simulink subsystem "PvtSubSys_VSM_ACC"  (R2020b)
settings: Solver=VariableStepAuto  StartTime=0.0  StopTime=10.0  RelTol=1e-3
values from neighbouring files (symbols this model uses):
  P_VSM_ACC_AutoGoSW = 1.0    [ACC.sldd]
  P_VSM_ACC_BOMEntry_ACCDecReqValue = -0.5    [ACC.sldd]
  P_VSM_ACC_BOMEntry_AxvRefMs2 = -0.5    [ACC.sldd]
  P_VSM_ACC_BOMExit_ACCDecReqValue = -0.3    [ACC.sldd]
  P_VSM_ACC_BrakeOnlyNum = 500.0    [ACC.sldd]
  P_VSM_ACC_RadarOffset = 0.5    [ACC.sldd]
  P_VSM_ACC_StandActiveNumACCMode = 1500.0    [ACC.sldd]
  P_VSM_ACC_StandActiveNumHWAMode = 1500.0    [ACC.sldd]
  P_VSM_ACCExit_AccOverride = 900.0    [ACC.sldd]
  P_VSM_ACCExit_StandWaitTime = 180.0    [ACC.sldd]
  P_VSM_TJA_ActiveWaitNum = 3000.0    [ACC.sldd]
undefined symbols (not defined in the file or in its folder): ACC_STATE, HWAError_Error, HWAError_ErrorBlindness, HWAError_ErrorFast, HWAError_Inhibit, P_Global_VehiclePowerType, P_VSM_PowerTrainConfig, TJA_STATE
libraries: simulink x136, TrueDurationTime x17
(part 1 of 2)
settings Model: Creator=GW00133806  LastModifiedBy=GW00201299

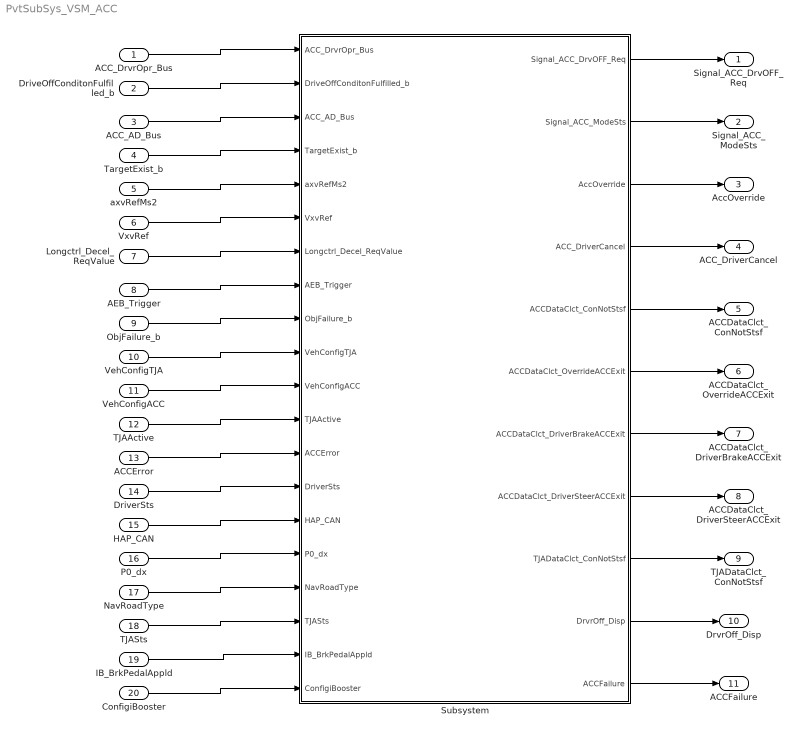
== system PvtSubSys_VSM_ACC ==
  ACC_DrvrOpr_Bus : Inport  OutDataTypeStr=Bus: ACC_DrvrOpr_Bus
  DriveOffConditonFulfilled_b : Inport  Port=2  OutDataTypeStr=boolean
  ACC_AD_Bus : Inport  Port=3
  TargetExist_b : Inport  Port=4  OutDataTypeStr=boolean
  axvRefMs2 : Inport  Port=5  OutDataTypeStr=single
  VxvRef : Inport  Port=6  OutDataTypeStr=single
  Longctrl_Decel_ReqValue : Inport  Port=7  OutDataTypeStr=single
  AEB_Trigger : Inport  Port=8  OutDataTypeStr=boolean
  ObjFailure_b : Inport  Port=9  OutDataTypeStr=boolean
  VehConfigTJA : Inport  Port=10  OutDataTypeStr=boolean
  VehConfigACC : Inport  Port=11  OutDataTypeStr=boolean
  TJAActive : Inport  Port=12  OutDataTypeStr=boolean
  ACCError : Inport  Port=13  OutDataTypeStr=uint8
  DriverSts : Inport  Port=14  OutDataTypeStr=uint8
  HAP_CAN : Inport  Port=15  OutDataTypeStr=Bus: HAP_CAN
  P0_dx : Inport  Port=16  OutDataTypeStr=single
  NavRoadType : Inport  Port=17  OutDataTypeStr=uint8
  TJASts : Inport  Port=18
  IB_BrkPedalAppld : Inport  Port=19
  ConfigiBooster : Inport  Port=20
  Subsystem : Subsystem
  Signal_ACC_DrvOFF_Req : Outport
  Signal_ACC_ModeSts : Outport  Port=2
  AccOverride : Outport  Port=3
  ACC_DriverCancel : Outport  Port=4
  ACCDataClct_ConNotStsf : Outport  Port=5
  ACCDataClct_OverrideACCExit : Outport  Port=6
  ACCDataClct_DriverBrakeACCExit : Outport  Port=7
  ACCDataClct_DriverSteerACCExit : Outport  Port=8
  TJADataClct_ConNotStsf : Outport  Port=9
  DrvrOff_Disp : Outport  Port=10
  ACCFailure : Outport  Port=11
  wires:
  ConfigiBooster/1 -> Subsystem/20(ConfigiBooster)
  IB_BrkPedalAppld/1 -> Subsystem/19(IB_BrkPedalAppld)
  NavRoadType/1 -> Subsystem/17(NavRoadType)
  Subsystem/9(TJADataClct_ConNotStsf) -> TJADataClct_ConNotStsf/1
  Subsystem/4(ACC_DriverCancel) -> ACC_DriverCancel/1
  Subsystem/6(ACCDataClct_OverrideACCExit) -> ACCDataClct_OverrideACCExit/1
  VxvRef/1 -> Subsystem/6(VxvRef)
  Subsystem/7(ACCDataClct_DriverBrakeACCExit) -> ACCDataClct_DriverBrakeACCExit/1
  TargetExist_b/1 -> Subsystem/4(TargetExist_b)
  TJAActive/1 -> Subsystem/12(TJAActive)
  Subsystem/8(ACCDataClct_DriverSteerACCExit) -> ACCDataClct_DriverSteerACCExit/1
  Longctrl_Decel_ReqValue/1 -> Subsystem/7(Longctrl_Decel_ReqValue)
  axvRefMs2/1 -> Subsystem/5(axvRefMs2)
  Subsystem/5(ACCDataClct_ConNotStsf) -> ACCDataClct_ConNotStsf/1
  VehConfigTJA/1 -> Subsystem/10(VehConfigTJA)
  Subsystem/1(Signal_ACC_DrvOFF_Req) -> Signal_ACC_DrvOFF_Req/1
  ACCError/1 -> Subsystem/13(ACCError)
  Subsystem/3(AccOverride) -> AccOverride/1
  VehConfigACC/1 -> Subsystem/11(VehConfigACC)
  Subsystem/2(Signal_ACC_ModeSts) -> Signal_ACC_ModeSts/1
  ObjFailure_b/1 -> Subsystem/9(ObjFailure_b)
  AEB_Trigger/1 -> Subsystem/8(AEB_Trigger)
  ACC_DrvrOpr_Bus/1 -> Subsystem/1(ACC_DrvrOpr_Bus)
  DriveOffConditonFulfilled_b/1 -> Subsystem/2(DriveOffConditonFulfilled_b)
  ACC_AD_Bus/1 -> Subsystem/3(ACC_AD_Bus)
  DriverSts/1 -> Subsystem/14(DriverSts)
  HAP_CAN/1 -> Subsystem/15(HAP_CAN)
  P0_dx/1 -> Subsystem/16(P0_dx)
  Subsystem/10(DrvrOff_Disp) -> DrvrOff_Disp/1
  Subsystem/11(ACCFailure) -> ACCFailure/1
  TJASts/1 -> Subsystem/18(TJASts)

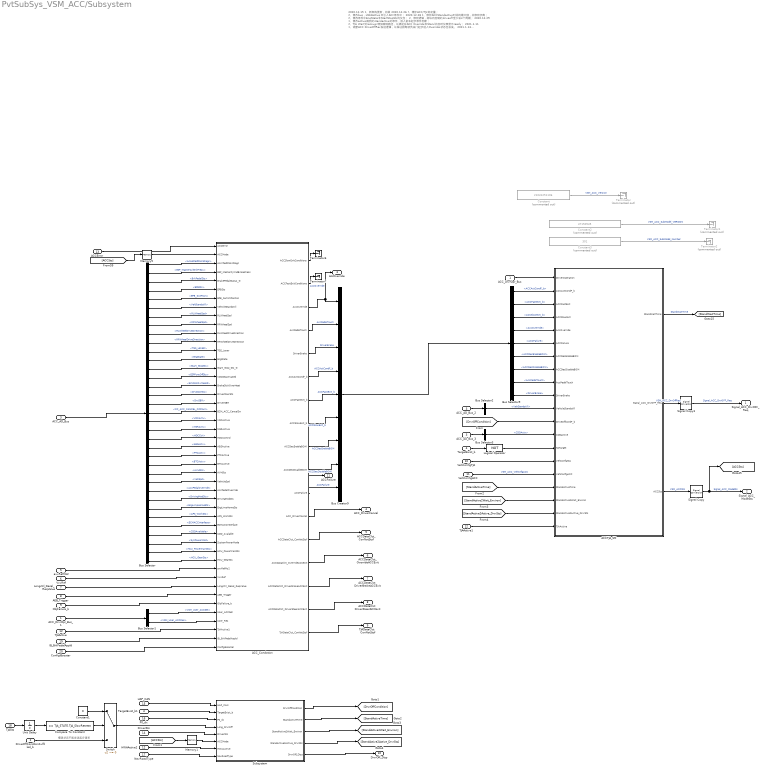
== system PvtSubSys_VSM_ACC/Subsystem ==
  note: 2020.12.15
      | 1、新架构更新，初版
      | 2020.12.26
      | 1、增加ACC/TJA标定量；
      | 2、修改bug，HWAActive未引入ACC条件中；
      | 2020.12.28
      | 1、修改ACCStandactive时间的最大值，并修改字典；
      | 2、修改条件中EngState和StartStopSts的交互；
      | 3、修改逻辑，给纵向控制的driveoff至少发3个周期；
      | 2020.12.29
      | 1、修改active跳到的standactive的条件，加入前车起步条件判断；
      | 2、TJA_Wait到recover增加跳转路径，以满足在ACC Override和Stand状态时仪表显示ready；
      | 2021.1.11
      | 1、调整ACC DriveOffReq发送逻辑，以保证因驾驶员油门起步进入Override状态也会发。
      | 2021.1.13
      | 添加基于驾驶员状态的自动起步逻辑，并用标定量默认关闭；
      | 2021.1.19
      | ACC起步条件增加；
      | 增加观测量；
      | 2021.1.23
      | TJA状态机修改；
      | 2021.1.25
      | ACC状态机中进入standactive的条件删去driveroff；
      | 2021.1.27
      | 1、TJA进入ready修改；
      | 2、ACCdriveroff修改；
      | 2021.1.30
      | TJA逻辑修改
      | 2021.2.1
      | ACC刹车&&standstill激活条件修改；
      | 2021.2.2
      | TJA override逻辑加入HWAActive判断；
      | 2021.2.3
      | TJAWait状态计时bug修改；
      | ACC发DrvrOff逻辑修改；
      | TJAActiveNum阈值修改为4；
      | 2021.2.4
      | DrvrOffReq输出逻辑修改；
      | 2021.2.5
      | ACC Passive状态重写TJAstopexit的值
      | 2021.2.7
      | 增加观测量Override退出条件；
      | 20210217
      | ACCError策略修改；
      | 20210219
      | 删去ACC的CDD和ECM导致的Error，因为在诊断里已经做了，报inhibit
      | 20210224
      | ACC启停条件修改：or2and；
      | 20210308
      | 删去状态机中起步HWA相关条件；
      | 2021.3.12
      | SafeStop置位延迟5s
      | 2021.3.15
      | ACC Override不退出TJA控制；
  note: 慢退状态不能发送起步请求
  ACC_DrvrOpr_Bus : Inport  OutDataTypeStr=Bus: ACC_DrvrOpr_Bus
  DriveOffConditonFulfilled_b : Inport  Port=2  OutDataTypeStr=boolean
  ACC_AD_Bus : Inport  Port=3
  TargetExist_b : Inport  Port=4  OutDataTypeStr=boolean
  axvRefMs2 : Inport  Port=5  OutDataTypeStr=single
  VxvRef : Inport  Port=6  OutDataTypeStr=single
  Longctrl_Decel_ReqValue : Inport  Port=7  OutDataTypeStr=single
  AEB_Trigger : Inport  Port=8  OutDataTypeStr=boolean
  ObjFailure_b : Inport  Port=9  OutDataTypeStr=boolean
  VehConfigTJA : Inport  Port=10  OutDataTypeStr=boolean
  VehConfigACC : Inport  Port=11  OutDataTypeStr=boolean
  TJAActive : Inport  Port=12  OutDataTypeStr=boolean
  ACCError : Inport  Port=13  OutDataTypeStr=uint8
  DriverSts : Inport  Port=14  OutDataTypeStr=uint8
  HAP_CAN : Inport  Port=15  OutDataTypeStr=Bus: HAP_CAN
  P0_dx : Inport  Port=16  OutDataTypeStr=single
  NavRoadType : Inport  Port=17
  TJASts : Inport  Port=18
  IB_BrkPedalAppld : Inport  Port=19
  ConfigiBooster : Inport  Port=20
  ACCTJA_SM : Subsystem
  ACC_AD_Bus_2 : InportShadow  Port=3
  ACC_AD_Bus_3 : InportShadow  Port=3
  ACC_Condotion : Subsystem
  ACC_DrvrOpr_Bus_1 : InportShadow  OutDataTypeStr=Bus: ACC_DrvrOpr_Bus
  Bus Creator9 : BusCreator  Inputs=9
  Bus Selector : BusSelector  OutputSignals=AccelPedlPosnDiagc,ESP_MasterCylBrkPress,BrkPedalSts,EPBSts,EPB_SwtPosn,VehStandstill,RLWheelSpd,RRWheelSpd,RLWheelDriveDirection,RRWheelDriveDirection,TGS_LEVER,EngState,Start_StopSts,ESPFuncOffSts,BrkDskOvrheatd,DrvDoorSts,DrvSBR,CC_ACC_CANCEL_OFFSwt,VDCActv,MSRActv,HDCCtrl,ABSActv,PTCActv,BTCActv,AVHSts,VehSpd,AccPedalOverride,DrivingModDis,EngLimpHomeSts,APS_WorkSts,ECMACCInterface,CDDAvailable,SysPowerMod,HCU_PowertrainSts,HCU_GearSts
  Bus Selector1 : BusSelector  OutputSignals=VSM_User_ACCSet,VSM_User_ACCRes
  Bus Selector2 : BusSelector  OutputSignals=VehStandstill
  Bus Selector3 : BusSelector  OutputSignals=CDDActv
  Bus Selector9 : BusSelector  OutputSignals=ACCActCondF_b,ACCFastExit_b,ACCSlowExit_b,AccOverride,ACCFailure,ACCDecEnableBOM,ACCDecDisableBOM,AccPedalTouch,DriverBrake
  Compare To Constant : simulink/Logic and Bit Operations/Compare To Constant  relop===  const=TJA_STATE.TJA_SlowRetreat  OutDataTypeStr=boolean
  Constant : Constant  Commented=on  Value=21031251106
  Constant1 : Constant  Value=0  OutDataTypeStr=boolean
  Constant2 : Constant  Commented=on  Value=37150535  OutDataTypeStr=uint32
  Constant3 : Constant  Commented=on  Value=301  OutDataTypeStr=uint16
  HWAActive2 : InportShadow  Port=12  OutDataTypeStr=boolean
  Logical Operator : Logic  Operator=NOT  AllPortsSameDT=off  OutDataTypeStr=boolean
  Memory1 : Memory  InitialCondition=ACC_STATE.ACC_Off  InheritSampleTime=on
  Memory5 : Memory  InitialCondition=ACC_STATE.ACC_Off  InheritSampleTime=on
  Signal Copy : SignalConversion  OverrideOpt=off
  Signal Copy3 : SignalConversion  OverrideOpt=off
  Subsystem : Subsystem
  Switch : Switch  Criteria=u2 ~= 0
  TJAActive1 : InportShadow  Port=12  OutDataTypeStr=boolean
  TargetExist_b1 : InportShadow  Port=4  OutDataTypeStr=boolean
  Terminator : Terminator  Commented=on
  Terminator1 : Terminator  Commented=on
  Terminator2 : Terminator  Commented=on
  Terminator6 : Terminator
  Terminator7 : Terminator
  Unit Delay : UnitDelay  InitialCondition=TJA_STATE.TJA_Off  SampleTime=-1  HasFrameUpgradeWarning=on
  Signal_ACC_DrvOFF_Req : Outport
  Signal_ACC_ModeSts : Outport  Port=2
  AccOverride : Outport  Port=3
  ACC_DriverCancel : Outport  Port=4
  ACCDataClct_ConNotStsf : Outport  Port=5
  ACCDataClct_OverrideACCExit : Outport  Port=6
  ACCDataClct_DriverBrakeACCExit : Outport  Port=7
  ACCDataClct_DriverSteerACCExit : Outport  Port=8
  TJADataClct_ConNotStsf : Outport  Port=9
  DrvrOff_Disp : Outport  Port=10
  ACCFailure : Outport  Port=11
  wires:
  Constant2/1 -> Terminator1/1  "VSM_ACC_SubModel_VERSION"
  Constant3/1 -> Terminator2/1  "VSM_ACC_SubModel_Number"
  Switch/1 -> Subsystem/4(Long_DrvrOff)
  Constant1/1 -> Switch/1
  Compare To Constant/1 -> Switch/2
  TJASts/1 -> Unit Delay/1
  TJAActive1/1 -> ACCTJA_SM/20(TJAActive)
  [StandActive2Active_DrvrSts] -> ACCTJA_SM/19(StandActive2Active_DrvrSts)
  [StandActive2Wait_Environ] -> ACCTJA_SM/18(StandActive2Wait_Environ)
  [StandActiveTime] -> ACCTJA_SM/17(StandActiveTime)
  Subsystem/5(DrvrOff_Disp) -> DrvrOff_Disp/1
  Subsystem/4(StandActive2Active_DrvrSts) -> [StandActive2Active_DrvrSts]
  Subsystem/3(StandActive2Wait_Environ) -> [StandActive2Wait_Environ]
  Subsystem/2(StandActiveTime) -> [StandActiveTime]
  NavRoadType/1 -> Subsystem/8(NavRoadType)
  HWAActive2/1 -> Subsystem/7(HWAActive)
  Memory1/1 -> Subsystem/6(ACCMode)
  DriverSts/1 -> Subsystem/5(DriverSts)
  [ACCSts] -> Memory1/1
  TargetExist_b1/1 -> Subsystem/2(TargetExist_b)
  P0_dx/1 -> Subsystem/3(P0_dx)
  [DrvrOffCondition] -> ACCTJA_SM/12(DriveOffCondF_b)
  Subsystem/1(DrvrOffCondition) -> [DrvrOffCondition]
  DriveOffConditonFulfilled_b/1 -> Switch/3
  HAP_CAN/1 -> Subsystem/1(HAP_CAN)
  Constant/1 -> Terminator/1  "VSM_ACC_Version"
  TJAActive/1 -> ACC_Condotion/45(TJAActive1)
  Bus Selector/11 -> ACC_Condotion/13(TGS_Lever)  "<TGS_LEVER>"
  ACC_Condotion/5(DriverBrake) -> Bus Creator9/3  "DriverBrake"
  Bus Selector/15 -> ACC_Condotion/17(BrakeDiskOverHeat)  "<BrkDskOvrheatd>"
  ACC_AD_Bus_3/1 -> Bus Selector3/1
  ACC_Condotion/1(ACCSlowExitConditions) -> Terminator6/1
  VxvRef/1 -> ACC_Condotion/39(VxvRef)
  Bus Selector/5 -> ACC_Condotion/7(EPB_SwtichPositon)  "<EPB_SwtPosn>"
  Bus Selector1/2 -> ACC_Condotion/44(User_Res)  "<VSM_User_ACCRes>"
  ACC_Condotion/6(ACCActCondF_b) -> Bus Creator9/4  "ACCActCondF_b"
  ACC_AD_Bus/1 -> Bus Selector/1
  ACC_Condotion/12(ACC_DriverCancel) -> ACC_DriverCancel/1
  ACC_DrvrOpr_Bus_1/1 -> Bus Selector1/1
  ACC_Condotion/11(ACCFailure) -> Bus Creator9/9, ACCFailure/1  "ACCFailure"
  ACC_Condotion/15(ACCDataClct_DriverBrakeACCExit) -> ACCDataClct_DriverBrakeACCExit/1
  VehConfigTJA/1 -> ACCTJA_SM/15(VehConfigTJA)
  ACC_DrvrOpr_Bus/1 -> ACCTJA_SM/1(DirverOperation)
  Bus Selector/26 -> ACC_Condotion/28(VehicleSpd)  "<VehSpd>"
  ACC_AD_Bus_2/1 -> Bus Selector2/1
  Bus Selector9/2 -> ACCTJA_SM/3(ACCFastExit)  "<ACCFastExit_b>"
  Bus Selector9/9 -> ACCTJA_SM/10(DriverBrake)  "<DriverBrake>"
  ObjFailure_b/1 -> ACC_Condotion/42(ObjFailure_b)
  Bus Selector/20 -> ACC_Condotion/22(MSRActive)  "<MSRActv>"
  Bus Selector/28 -> ACC_Condotion/30(DrivingModDis)  "<DrivingModDis>"
  ACC_Condotion/13(ACCDataClct_ConNotStsf) -> ACCDataClct_ConNotStsf/1
  Bus Selector/13 -> ACC_Condotion/15(Start_Stop_Sts_G)  "<Start_StopSts>"
  ACC_Condotion/17(TJADataClct_ConNotStsf) -> TJADataClct_ConNotStsf/1
  ACCTJA_SM/1(StandWaitTime) -> [StandWaitTime]  "StandWaitTime"
  Bus Creator9/1 -> Bus Selector9/1
  Bus Selector2/1 -> ACCTJA_SM/11(VehicleStandstill)  "<VehStandstill>"
  Bus Selector/17 -> ACC_Condotion/19(DriverSBR)  "<DrvSBR>"
  Signal Copy3/1 -> Signal_ACC_DrvOFF_Req/1  "Signal_ACC_DrvOFF_Req"
  Bus Selector3/1 -> ACCTJA_SM/13(CDDactive)  "<CDDActv>"
  Longctrl_Decel_ReqValue/1 -> ACC_Condotion/40(Longctrl_Decel_ReqValue)
  Bus Selector/3 -> ACC_Condotion/5(BrakePedalStatus_G)  "<BrkPedalSts>"
  AEB_Trigger/1 -> ACC_Condotion/41(AEB_Trigger)
  Bus Selector9/8 -> ACCTJA_SM/9(AccPedalTouch)  "<AccPedalTouch>"
  VehConfigACC/1 -> ACCTJA_SM/16(VehConfigACC)  "VSM_ACC_VehCnfgACC"
  Bus Selector/2 -> ACC_Condotion/4(ESP_MasterCylindBrakePress)  "<ESP_MasterCylBrkPress>"
  Bus Selector/21 -> ACC_Condotion/23(HDCControl)  "<HDCCtrl>"
  Bus Selector/23 -> ACC_Condotion/25(PTCActive)  "<PTCActv>"
  ACC_Condotion/10(ACCDecDisableBOM) -> Bus Creator9/8  "ACCDecDisableBOM"
  ACC_Condotion/14(ACCDataClct_OverrideACCExit) -> ACCDataClct_OverrideACCExit/1
  Bus Selector/30 -> ACC_Condotion/32(APS_WorkSts)  "<APS_WorkSts>"
  Bus Selector/12 -> ACC_Condotion/14(EngState)  "<EngState>"
  ACC_Condotion/3(AccOverride) -> Bus Creator9/1, AccOverride/1  "AccOverride"
  Signal Copy/1 -> [ACCSts], Signal_ACC_ModeSts/1  "Signal_ACC_ModeSts"
  Bus Selector/29 -> ACC_Condotion/31(EngLimpHomeSts)  "<EngLimpHomeSts>"
  axvRefMs2/1 -> ACC_Condotion/38(axvRefMs2)
  Bus Selector/22 -> ACC_Condotion/24(ABSActive)  "<ABSActv>"
  ACCError/1 -> ACC_Condotion/1(ACCError)
  Memory5/1 -> ACC_Condotion/2(ACCMode)
  Bus Selector/14 -> ACC_Condotion/16(VDCDeactivated)  "<ESPFuncOffSts>"
  Bus Selector/10 -> ACC_Condotion/12(RRWheelDriveDirection)  "<RRWheelDriveDirection>"
  ACC_Condotion/9(ACCDecEnableBOM) -> Bus Creator9/7  "ACCDecEnableBOM"
  Bus Selector/4 -> ACC_Condotion/6(EPBSts)  "<EPBSts>"
  TargetExist_b/1 -> Logical Operator/1
  ACC_Condotion/4(AccPedalTouch) -> Bus Creator9/2  "AccPedalTouch"
  Bus Selector/27 -> ACC_Condotion/29(AccPedalOverride)  "<AccPedalOverride>"
  ACC_Condotion/16(ACCDataClct_DriverSteerACCExit) -> ACCDataClct_DriverSteerACCExit/1
  Bus Selector/24 -> ACC_Condotion/26(BTCActive)  "<BTCActv>"
  Bus Selector/7 -> ACC_Condotion/9(RLWheelSpd)  "<RLWheelSpd>"
  Bus Selector/18 -> ACC_Condotion/20(ECM_ACC_CancelSw)  "<CC_ACC_CANCEL_OFFSwt>"
  ACC_Condotion/8(ACCSlowExit_b) -> Bus Creator9/6  "ACCSlowExit_b"
  [ACCSts] -> Memory5/1
  Bus Selector9/6 -> ACCTJA_SM/7(ACCDecEnableBOM)  "<ACCDecEnableBOM>"
  Bus Selector1/1 -> ACC_Condotion/43(User_ACCSet)  "<VSM_User_ACCSet>"
  Bus Selector9/3 -> ACCTJA_SM/4(ACCSlowExit)  "<ACCSlowExit_b>"
  Bus Selector9/4 -> ACCTJA_SM/5(AccOverride)  "<AccOverride>"
  Bus Selector/8 -> ACC_Condotion/10(RRWheelSpd)  "<RRWheelSpd>"
  ACC_Condotion/2(ACCFastExitConditions) -> Terminator7/1
  ACC_Condotion/7(ACCFastExit_b) -> Bus Creator9/5  "ACCFastExit_b"
  Bus Selector9/7 -> ACCTJA_SM/8(ACCDecDisableBOM)  "<ACCDecDisableBOM>"
  Bus Selector/31 -> ACC_Condotion/33(ECMACCInterface)  "<ECMACCInterface>"
  Bus Selector/19 -> ACC_Condotion/21(VDCActive)  "<VDCActv>"
  Logical Operator/1 -> ACCTJA_SM/14(NoTarget)
  Bus Selector/25 -> ACC_Condotion/27(AVHSts)  "<AVHSts>"
  Bus Selector/16 -> ACC_Condotion/18(DriverDoorSts)  "<DrvDoorSts>"
  Bus Selector/6 -> ACC_Condotion/8(VehicleStandstill)  "<VehStandstill>"
  Bus Selector9/5 -> ACCTJA_SM/6(ACCFailure)  "<ACCFailure>"
  Bus Selector9/1 -> ACCTJA_SM/2(ACCActCondF_b)  "<ACCActCondF_b>"
  Bus Selector/33 -> ACC_Condotion/35(SystemPowerMode)  "<SysPowerMod>"
  Bus Selector/9 -> ACC_Condotion/11(RLWheelDriveDirection)  "<RLWheelDriveDirection>"
  Bus Selector/1 -> ACC_Condotion/3(AccrPedlPosnDiagc)  "<AccelPedlPosnDiagc>"
  Bus Selector/32 -> ACC_Condotion/34(CDD_Avalable)  "<CDDAvailable>"
  ACCTJA_SM/3(ACCSts) -> Signal Copy/1  "VSM_ACCSts"
  ACCTJA_SM/2(Signal_ACC_DrvOFF_Req) -> Signal Copy3/1  "VSM_ACC_DrvOffReq"
  Unit Delay/1 -> Compare To Constant/1
  Bus Selector/34 -> ACC_Condotion/36(HCU_PowertrainSts)  "<HCU_PowertrainSts>"
  Bus Selector/35 -> ACC_Condotion/37(HCU_GearSts)  "<HCU_GearSts>"
  IB_BrkPedalAppld/1 -> ACC_Condotion/46(IB_BrkPedalAppld)
  ConfigiBooster/1 -> ACC_Condotion/47(ConfigiBooster)

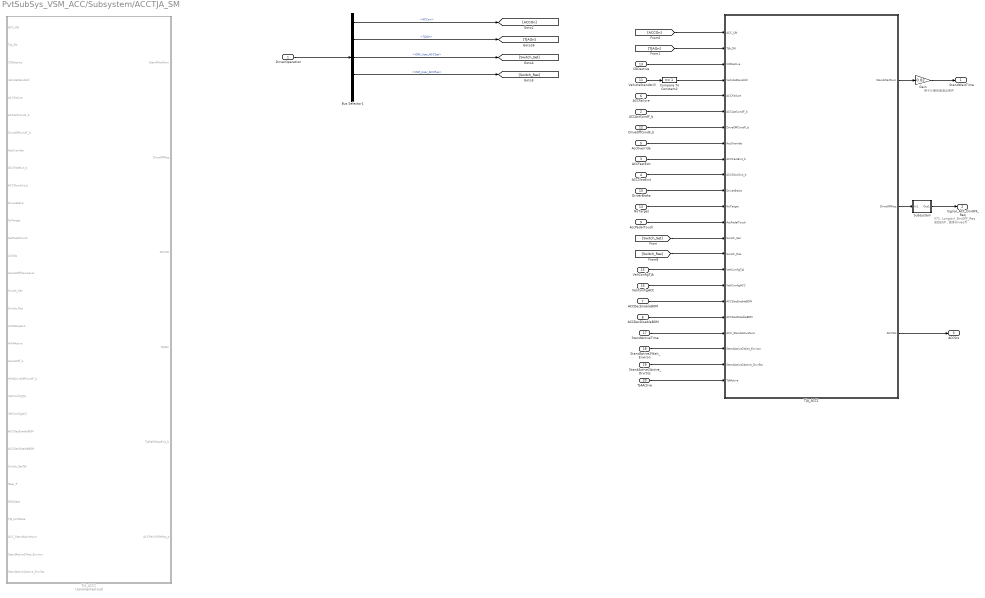
== system PvtSubSys_VSM_ACC/Subsystem/ACCTJA_SM ==
  note: V71: Longctrl_DrvOFF_Req
      | 发给ESP，请求dirveoff
  note: 用于计算快速退出条件
  DirverOperation : Inport
  ACCActCondF_b : Inport  Port=2
  ACCFastExit : Inport  Port=3
  ACCSlowExit : Inport  Port=4
  AccOverride : Inport  Port=5
  ACCFailure : Inport  Port=6
  ACCDecEnableBOM : Inport  Port=7
  ACCDecDisableBOM : Inport  Port=8
  AccPedalTouch : Inport  Port=9
  DriverBrake : Inport  Port=10
  VehicleStandstill : Inport  Port=11
  DriveOffCondF_b : Inport  Port=12
  CDDactive : Inport  Port=13
  NoTarget : Inport  Port=14
  VehConfigTJA : Inport  Port=15
  VehConfigACC : Inport  Port=16
  StandActiveTime : Inport  Port=17
  StandActive2Wait_Environ : Inport  Port=18
  StandActive2Active_DrvrSts : Inport  Port=19
  TJAActive : Inport  Port=20
  Bus Selector1 : BusSelector  OutputSignals=ACCon,TJAOn,VSM_User_ACCSet,VSM_User_ACCRes,VSM_User_TJASet
  Compare To Constant2 : simulink/Logic and Bit Operations/Compare To Constant  relop===  const=1  OutDataTypeStr=boolean
  Gain : Gain  Gain=0.02  ParamDataTypeStr=uint16  OutDataTypeStr=uint16
  Subsystem : Subsystem
  TJA_ACC1 : Stateflow chart  TreatAsAtomicUnit=on
  TJA_ACC2 : Stateflow chart  Commented=on  TreatAsAtomicUnit=on
  StandWaitTime : Outport  OutDataTypeStr=uint16
  Signal_ACC_DrvOFF_Req : Outport  Port=2  OutDataTypeStr=boolean
  ACCSts : Outport  Port=3
  wires:
  TJAActive/1 -> TJA_ACC1/23(TJAActive)
  StandActive2Active_DrvrSts/1 -> TJA_ACC1/22(StandActive2Active_DrvrSts)
  StandActive2Wait_Environ/1 -> TJA_ACC1/21(StandActive2Wait_Environ)
  StandActiveTime/1 -> TJA_ACC1/20(ACC_StandActiveNum)
  Subsystem/1(Out1) -> Signal_ACC_DrvOFF_Req/1
  TJA_ACC1/2(DriveOffReq) -> Subsystem/1(In1)
  VehicleStandstill/1 -> Compare To Constant2/1
  Bus Selector1/4 -> [Switch_Res]  "<VSM_User_ACCRes>"
  Bus Selector1/3 -> [Switch_Set]  "<VSM_User_ACCSet>"
  Bus Selector1/2 -> [TJAOn]  "<TJAOn>"
  Bus Selector1/1 -> [ACCOn]  "<ACCon>"
  DirverOperation/1 -> Bus Selector1/1
  ACCDecDisableBOM/1 -> TJA_ACC1/19(ACCDecDisableBOM)
  ACCDecEnableBOM/1 -> TJA_ACC1/18(ACCDecEnableBOM)
  VehConfigACC/1 -> TJA_ACC1/17(VehConfigACC)
  VehConfigTJA/1 -> TJA_ACC1/16(VehConfigTJA)
  TJA_ACC1/3(ACCSts) -> ACCSts/1
  [Switch_Res] -> TJA_ACC1/15(Switch_Res)
  [Switch_Set] -> TJA_ACC1/14(Switch_Set)
  TJA_ACC1/1(StandWaitNum) -> Gain/1
  AccPedalTouch/1 -> TJA_ACC1/13(AccPedalTouch)
  NoTarget/1 -> TJA_ACC1/12(NoTarget)
  DriverBrake/1 -> TJA_ACC1/11(DriverBrake)
  ACCSlowExit/1 -> TJA_ACC1/10(ACCSlowExit_b)
  ACCFastExit/1 -> TJA_ACC1/9(ACCFastExit_b)
  AccOverride/1 -> TJA_ACC1/8(AccOverride)
  DriveOffCondF_b/1 -> TJA_ACC1/7(DriveOffCondF_b)
  ACCActCondF_b/1 -> TJA_ACC1/6(ACCActCondF_b)
  ACCFailure/1 -> TJA_ACC1/5(ACCFailure)
  CDDactive/1 -> TJA_ACC1/3(CDDactive)
  Compare To Constant2/1 -> TJA_ACC1/4(VehicleStandstill)
  [TJAOn] -> TJA_ACC1/2(TJA_ON)
  [ACCOn] -> TJA_ACC1/1(ACC_ON)
  Gain/1 -> StandWaitTime/1

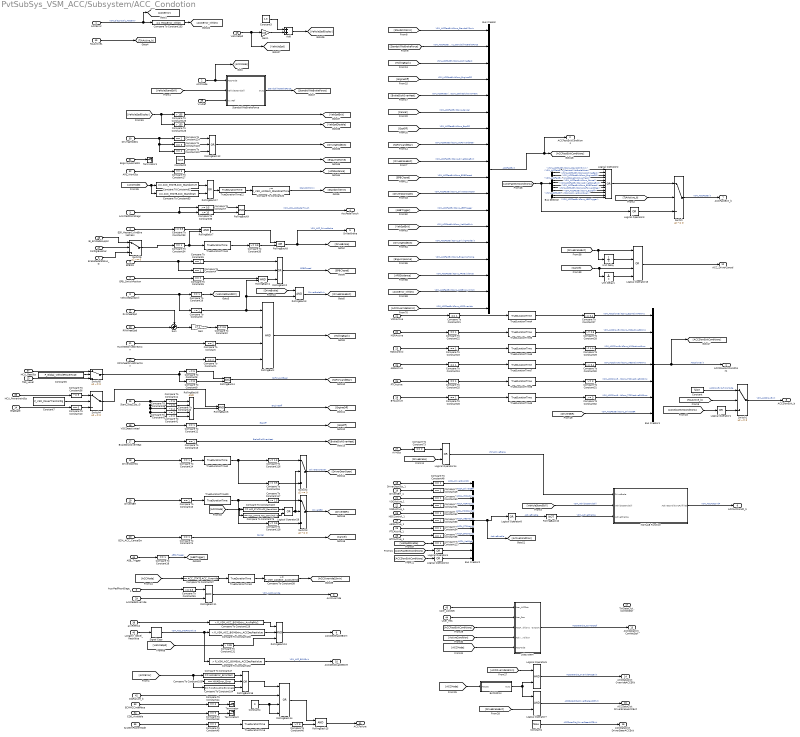
== system PvtSubSys_VSM_ACC/Subsystem/ACC_Condotion ==
  ACCError : Inport
  ACCMode : Inport  Port=2
  AccrPedlPosnDiagc : Inport  Port=3
  ESP_MasterCylindBrakePress : Inport  Port=4
  BrakePedalStatus_G : Inport  Port=5
  EPBSts : Inport  Port=6
  EPB_SwtichPositon : Inport  Port=7
  VehicleStandstill : Inport  Port=8
  RLWheelSpd : Inport  Port=9
  RRWheelSpd : Inport  Port=10
  RLWheelDriveDirection : Inport  Port=11
  RRWheelDriveDirection : Inport  Port=12
  TGS_Lever : Inport  Port=13
  EngState : Inport  Port=14
  Start_Stop_Sts_G : Inport  Port=15
  VDCDeactivated : Inport  Port=16
  BrakeDiskOverHeat : Inport  Port=17
  DriverDoorSts : Inport  Port=18
  DriverSBR : Inport  Port=19
  ECM_ACC_CancelSw : Inport  Port=20
  VDCActive : Inport  Port=21
  MSRActive : Inport  Port=22
  HDCControl : Inport  Port=23
  ABSActive : Inport  Port=24
  PTCActive : Inport  Port=25
  BTCActive : Inport  Port=26
  AVHSts : Inport  Port=27
  VehicleSpd : Inport  Port=28
  AccPedalOverride : Inport  Port=29
  DrivingModDis : Inport  Port=30
  EngLimpHomeSts : Inport  Port=31
  APS_WorkSts : Inport  Port=32
  ECMACCInterface : Inport  Port=33
  CDD_Avalable : Inport  Port=34
  SystemPowerMode : Inport  Port=35
  HCU_PowertrainSts : Inport  Port=36
  HCU_GearSts : Inport  Port=37
  axvRefMs2 : Inport  Port=38
  VxvRef : Inport  Port=39
  Longctrl_Decel_ReqValue : Inport  Port=40
  AEB_Trigger : Inport  Port=41
  ObjFailure_b : Inport  Port=42
  User_ACCSet : Inport  Port=43
  User_Res : Inport  Port=44
  TJAActive1 : Inport  Port=45
  IB_BrkPedalAppld : Inport  Port=46
  ConfigiBooster : Inport  Port=47
  ABSActive_1 : InportShadow  Port=24
  AccrPedlPosnDiagc_1 : InportShadow  Port=3
  Add : Sum
  BTCActive_1 : InportShadow  Port=26
  Bus Selector : BusSelector  OutputSignals=VSM_ACCFastExitCons_Standstill3min,VSM_ACCFastExitCons_StandstillNoBrakeForce,VSM_ACCFastExitCons_RollingBack,VSM_ACCFastExitCons_EngineOff,VSM_ACCFastExitCons_BrakeDiskOverHeat,VSM_ACCFastExitCons_Cancel,VSM_ACCFastExitCons_DriveBrakeExit,VSM_ACCFastExitCons_EPBClosed,VSM_ACCFastExitCons_NoForwardGear,VSM_ACCFastExitCons_EspOff,VSM_ACCFastExitCons_DriverDoorOpen,VSM_ACCFastExitCons_AEBTrigger
  Bus Creator : BusCreator  Inputs=18
  Bus Creator1 : BusCreator  Inputs=7
  Bus Creator2 : BusCreator  Inputs=11
  Compare To Constant{,1,5..6,45,73,124} (7 alike) : simulink/Logic and Bit Operations/Compare To Constant  relop===  const=2  OutDataTypeStr=boolean
  Compare To Constant10 : simulink/Logic and Bit Operations/Compare To Constant  relop===  const=0  OutDataTypeStr=boolean
  Compare To Constant103 : simulink/Logic and Bit Operations/Compare To Constant  relop===  const=HWAError_Error  OutDataTypeStr=boolean
  Compare To Constant104 : simulink/Logic and Bit Operations/Compare To Constant  relop===  const=HWAError_ErrorBlindness  OutDataTypeStr=boolean
  Compare To Constant11 : simulink/Logic and Bit Operations/Compare To Constant  relop=~=  const=6  OutDataTypeStr=boolean
  Compare To Constant116 : simulink/Logic and Bit Operations/Compare To Constant  relop=>=  const=1.5  OutDataTypeStr=boolean
  Compare To Constant117 : simulink/Logic and Bit Operations/Compare To Constant  relop=>=  const=1.5  OutDataTypeStr=boolean
  Compare To Constant{7,16,33,35,61,118} (6 alike) : simulink/Logic and Bit Operations/Compare To Constant  relop=>=  const=0.5  OutDataTypeStr=boolean
  Compare To Constant119 : simulink/Logic and Bit Operations/Compare To Constant  relop===  const=ACC_STATE.ACC_StandWait  OutDataTypeStr=boolean
  Compare To Constant{4,12..15,18..19,21..26,34,48..55,74,127} (24 alike) : simulink/Logic and Bit Operations/Compare To Constant  relop===  const=1  OutDataTypeStr=boolean
  Compare To Constant122 : simulink/Logic and Bit Operations/Compare To Constant  relop===  const=4  OutDataTypeStr=boolean
  Compare To Constant123 : simulink/Logic and Bit Operations/Compare To Constant  relop===  const=3  OutDataTypeStr=boolean
  Compare To Constant125 : simulink/Logic and Bit Operations/Compare To Constant  relop=>  const=155  OutDataTypeStr=boolean
  Compare To Constant126 : simulink/Logic and Bit Operations/Compare To Constant  relop=>  const=150  OutDataTypeStr=boolean
  Compare To Constant129 : simulink/Logic and Bit Operations/Compare To Constant  relop=<  const=P_VSM_ACC_BOMEntry_AxvRefMs2  OutDataTypeStr=boolean
  Compare To Constant130 : simulink/Logic and Bit Operations/Compare To Constant  relop=<  const=P_VSM_ACC_BOMEntry_ACCDecReqValue  OutDataTypeStr=boolean
  Compare To Constant131 : simulink/Logic and Bit Operations/Compare To Constant  relop=>  const=0.36  OutDataTypeStr=boolean
  Compare To Constant132 : simulink/Logic and Bit Operations/Compare To Constant  relop=>  const=P_VSM_ACC_BOMExit_ACCDecReqValue  OutDataTypeStr=boolean
  Compare To Constant133 : simulink/Logic and Bit Operations/Compare To Constant  relop===  const=HWAError_Inhibit  OutDataTypeStr=boolean
  Compare To Constant17 : simulink/Logic and Bit Operations/Compare To Constant  relop===  const=3  OutDataTypeStr=boolean
  Compare To Constant2 : simulink/Logic and Bit Operations/Compare To Constant  relop=>=  const=0.6  OutDataTypeStr=boolean
  Compare To Constant20 : simulink/Logic and Bit Operations/Compare To Constant  relop=>=  const=P_VSM_ACCExit_StandWaitTime  OutDataTypeStr=boolean
  Compare To Constant27 : simulink/Logic and Bit Operations/Compare To Constant  relop=>=  const=0.4  OutDataTypeStr=boolean
  Compare To Constant28 : simulink/Logic and Bit Operations/Compare To Constant  relop=>=  const=0.8  OutDataTypeStr=boolean
  Compare To Constant29 : simulink/Logic and Bit Operations/Compare To Constant  relop=>=  const=0.04  OutDataTypeStr=boolean
  Compare To Constant3 : simulink/Logic and Bit Operations/Compare To Constant  relop=~=  const=1  OutDataTypeStr=boolean
  Compare To Constant30 : simulink/Logic and Bit Operations/Compare To Constant  relop=>=  const=0.4  OutDataTypeStr=boolean
  Compare To Constant31 : simulink/Logic and Bit Operations/Compare To Constant  relop=>=  const=3  OutDataTypeStr=boolean
  Compare To Constant32 : simulink/Logic and Bit Operations/Compare To Constant  relop=>=  const=3  OutDataTypeStr=boolean
  Compare To Constant36 : simulink/Logic and Bit Operations/Compare To Constant  relop=<=  const=10  OutDataTypeStr=boolean
  Compare To Constant37 : simulink/Logic and Bit Operations/Compare To Constant  relop===  const=ACC_STATE.ACC_Override  OutDataTypeStr=boolean
  Compare To Constant38 : simulink/Logic and Bit Operations/Compare To Constant  relop=>=  const=P_VSM_ACCExit_AccOverride  OutDataTypeStr=boolean
  Compare To Constant39 : simulink/Logic and Bit Operations/Compare To Constant  relop=~=  const=5  OutDataTypeStr=boolean
  Compare To Constant40 : simulink/Logic and Bit Operations/Compare To Constant  relop=~=  const=4  OutDataTypeStr=boolean
  Compare To Constant41 : simulink/Logic and Bit Operations/Compare To Constant  relop=~=  const=3  OutDataTypeStr=boolean
  Compare To Constant42 : simulink/Logic and Bit Operations/Compare To Constant  relop=~=  const=2  OutDataTypeStr=boolean
  Compare To Constant43 : simulink/Logic and Bit Operations/Compare To Constant  relop===  const=0  OutDataTypeStr=boolean
  Compare To Constant44 : simulink/Logic and Bit Operations/Compare To Constant  relop===  const=0  OutDataTypeStr=boolean
  Compare To Constant46 : simulink/Logic and Bit Operations/Compare To Constant  relop=>=  const=6  OutDataTypeStr=boolean
  Compare To Constant47 : simulink/Logic and Bit Operations/Compare To Constant  relop===  const=HWAError_ErrorFast  OutDataTypeStr=boolean
  Compare To Constant56 : simulink/Logic and Bit Operations/Compare To Constant  relop=~=  const=5  OutDataTypeStr=boolean
  Compare To Constant62 : simulink/Logic and Bit Operations/Compare To Constant  relop===  const=ACC_STATE.ACC_StandActive  OutDataTypeStr=boolean
  Compare To Constant63 : simulink/Logic and Bit Operations/Compare To Constant  relop===  const=ACC_STATE.ACC_StandWait  OutDataTypeStr=boolean
  Compare To Constant75 : simulink/Logic and Bit Operations/Compare To Constant  relop===  const=ACC_STATE.ACC_StandActive  OutDataTypeStr=boolean
  Compare To Constant8 : simulink/Logic and Bit Operations/Compare To Constant  relop=~=  const=5  OutDataTypeStr=boolean
  Compare To Constant9 : simulink/Logic and Bit Operations/Compare To Constant  relop=~=  const=8  OutDataTypeStr=boolean
  Constant : Constant  Value=false
  Constant1 : Constant  Value=false
  Constant2 : Constant  Value=false
  Constant3 : Constant  Value=1.3
  Constant4 : Constant  Value=0  OutDataTypeStr=boolean
  Constant5 : Constant  Value=P_Global_VehiclePowerType
  Constant7 : Constant  Value=P_VSM_PowerTrainConfig
  DriverDoorSts_1 : InportShadow  Port=18
  DriverSBR_1 : InportShadow  Port=19
  Exit100ms : Subsystem
  Gain : Gain  Gain=1/7.2
  Gain1 : Gain  Gain=1.03
  HDCControl_1 : InportShadow  Port=23
  Logical Operator28 : Logic  Operator=OR  AllPortsSameDT=off  OutDataTypeStr=boolean
  Logical Operator6 : Logic  AllPortsSameDT=off  OutDataTypeStr=boolean
  Logical Operator7 : Logic  AllPortsSameDT=off  OutDataTypeStr=boolean
  Logical Operator{1,3..4,8,10} (5 alike) : Logic  Operator=OR  Inputs=1  AllPortsSameDT=off  OutDataTypeStr=boolean
  Logical Operator14 : Logic  Operator=OR  AllPortsSameDT=off  OutDataTypeStr=boolean
  Logical Operator15 : Logic  Operator=OR  Inputs=4  AllPortsSameDT=off  OutDataTypeStr=boolean
  Logical Operator2 : Logic  Operator=OR  Inputs=12  AllPortsSameDT=off  OutDataTypeStr=boolean
  MATLAB Function : MATLAB Function  TreatAsAtomicUnit=on
  MSRActive_1 : InportShadow  Port=22
  PTCActive_1 : InportShadow  Port=25
  RollingBack : Logic  Inputs=4  AllPortsSameDT=off  OutDataTypeStr=boolean
  RollingBack{1,3..5,7,9,11,15} (8 alike) : Logic  AllPortsSameDT=off  OutDataTypeStr=boolean
  RollingBack10 : Logic  Operator=NOT  Inputs=6  AllPortsSameDT=off  OutDataTypeStr=boolean
  RollingBack12 : Logic  Operator=OR  Inputs=3  AllPortsSameDT=off  OutDataTypeStr=boolean
  RollingBack13 : Logic  Inputs=3  AllPortsSameDT=off  OutDataTypeStr=boolean
  RollingBack14 : Logic  Operator=OR  Inputs=4  AllPortsSameDT=off  OutDataTypeStr=boolean
  RollingBack16 : Logic  Operator=OR  Inputs=3  AllPortsSameDT=off  OutDataTypeStr=boolean
  RollingBack17 : Logic  Operator=OR  AllPortsSameDT=off  OutDataTypeStr=boolean
  RollingBack2 : Logic  Operator=OR  Inputs=3  AllPortsSameDT=off  OutDataTypeStr=boolean
  RollingBack6 : Logic  Inputs=5  AllPortsSameDT=off  OutDataTypeStr=boolean
  RollingBack8 : Logic  Operator=OR  AllPortsSameDT=off  OutDataTypeStr=boolean
  Signal Copy : SignalConversion  OverrideOpt=off
  StandstillNoBrakeForce : Subsystem
  Subsystem : Subsystem
  Sum : Sum  Inputs=++|
  Switch{,1..6} (7 alike) : Switch  Criteria=u2 ~= 0
  Terminator : Terminator
  Terminator1 : Terminator
  Terminator2 : Terminator
  TrueDurationTime{,1..9,12,20} (12 alike) : TrueDurationTime/TrueDurationTime  TCycle=0.02
  Unit Delay : UnitDelay  SampleTime=-1  HasFrameUpgradeWarning=on
  Unit Delay1 : UnitDelay  SampleTime=-1  HasFrameUpgradeWarning=on
  VDCActive_1 : InportShadow  Port=21
  ACCSlowExitConditions : Outport
  ACCFastExitConditions : Outport  Port=2
  AccOverride : Outport  Port=3
  AccPedalTouch : Outport  Port=4
  DriverBrake : Outport  Port=5
  ACCActCondF_b : Outport  Port=6
  ACCFastExit_b : Outport  Port=7
  ACCSlowExit_b : Outport  Port=8
  ACCDecEnableBOM : Outport  Port=9
  ACCDecDisableBOM : Outport  Port=10
  ACCFailure : Outport  Port=11
  ACC_DriverCancel : Outport  Port=12
  ACCDataClct_ConNotStsf : Outport  Port=13
  ACCDataClct_OverrideACCExit : Outport  Port=14
  ACCDataClct_DriverBrakeACCExit : Outport  Port=15
  ACCDataClct_DriverSteerACCExit : Outport  Port=16
  TJADataClct_ConNotStsf : Outport  Port=17
  wires:
  Bus Selector/12 -> Logical Operator2/12  "<VSM_ACCFastExitCons_AEBTrigger>"
  Bus Selector/11 -> Logical Operator2/11  "<VSM_ACCFastExitCons_DriverDoorOpen>"
  Bus Selector/10 -> Logical Operator2/10  "<VSM_ACCFastExitCons_EspOff>"
  Bus Selector/9 -> Logical Operator2/9  "<VSM_ACCFastExitCons_NoForwardGear>"
  Bus Selector/8 -> Logical Operator2/8  "<VSM_ACCFastExitCons_EPBClosed>"
  Bus Selector/7 -> Logical Operator2/7  "<VSM_ACCFastExitCons_DriveBrakeExit>"
  Constant4/1 -> RollingBack14/3, RollingBack14/4
  Compare To Constant43/1 -> Terminator2/1
  Compare To Constant44/1 -> Terminator/1
  Logical Operator14/1 -> MATLAB Function/1(DriveBrake)  "VSM_DriveBrake"
  Signal Copy/1 -> Compare To Constant132/1, Compare To Constant130/1  "VSM_ACC_DecReqValue"
  Compare To Constant63/1 -> RollingBack17/2
  Compare To Constant62/1 -> RollingBack17/1
  TrueDurationTime12/1 -> Compare To Constant20/1
  RollingBack17/1 -> TrueDurationTime12/1
  [ACCMode] -> Compare To Constant62/1, Compare To Constant63/1
  RollingBack14/1 -> RollingBack15/1
  SystemPowerMode/1 -> Compare To Constant45/1
  TrueDurationTime/1 -> Compare To Constant46/1
  ECMACCInterface/1 -> Compare To Constant44/1
  RollingBack15/1 -> ACCFailure/1
  Compare To Constant45/1 -> TrueDurationTime/1
  Compare To Constant46/1 -> RollingBack15/2
  [ACCError] -> Compare To Constant47/1, Compare To Constant103/1, Compare To Constant104/1
  Compare To Constant103/1 -> RollingBack16/2
  CDD_Avalable/1 -> Compare To Constant43/1
  Compare To Constant47/1 -> RollingBack16/1
  ObjFailure_b/1 -> RollingBack14/2
  RollingBack16/1 -> RollingBack14/1
  Compare To Constant104/1 -> RollingBack16/3
  Compare To Constant42/1 -> RollingBack6/5
  Compare To Constant41/1 -> RollingBack6/4
  Compare To Constant40/1 -> RollingBack6/3
  Compare To Constant39/1 -> RollingBack6/2
  Compare To Constant11/1 -> RollingBack6/1
  TJAActive1/1 -> [TJAActive_b]
  [Standstill3min] -> Bus Creator/1  "VSM_ACCFastExitCons_Standstill3min"
  Compare To Constant34/1 -> TrueDurationTime1/1, RollingBack7/2
  Compare To Constant126/1 -> [VehSpdDisable]
  Compare To Constant26/1 -> TrueDurationTime9/1
  [ACCOverride15min] -> Bus Creator/18  "VSM_ACCFastExitCons_ACCOverride"
  Compare To Constant3/1 -> RollingBack/1, RollingBack3/2, RollingBack1/2
  Logical Operator4/1 -> Bus Creator2/10
  [ACCFastExitConditions] -> Logical Operator3/1, Bus Selector/1
  RollingBack6/1 -> RollingBack5/2
  Compare To Constant119/1 -> Logical Operator28/1
  Constant/1 -> Switch1/1  "AccSlowExit_HWAMode"
  [APSGuidance] -> Bus Creator/16  "VSM_ACCFastExitCons_APSGuidance"
  Bus Selector/3 -> Logical Operator2/3  "<VSM_ACCFastExitCons_RollingBack>"
  EngLimpHomeSts/1 -> Terminator1/1
  [ACCMode] -> Compare To Constant75/1, Compare To Constant119/1
  TrueDurationTime2/1 -> Compare To Constant16/1, Compare To Constant116/1
  APS_WorkSts/1 -> Compare To Constant17/1
  TrueDurationTime4/1 -> Compare To Constant27/1
  Constant3/1 -> Add/1
  VDCDeactivated/1 -> Compare To Constant12/1
  Constant2/1 -> [EngLimpHome]
  TrueDurationTime8/1 -> Compare To Constant31/1
  Add/1 -> [VehicleSpdDisplay]
  BTCActive_1/1 -> Compare To Constant55/1
  Compare To Constant55/1 -> Bus Creator2/8  "ACCA_BTCActive"
  TrueDurationTime3/1 -> Compare To Constant38/1
  Compare To Constant31/1 -> Bus Creator1/5  "VSM_ACCSlowExitCons_TCS1active3000ms"
  ACCMode/1 -> [ACCMode], StandstillNoBrakeForce/1(ACCMode)
  VehicleStandstill/1 -> Compare To Constant19/1, Compare To Constant3/1
  Compare To Constant9/1 -> RollingBack4/2
  Compare To Constant125/1 -> [VehSpdExit]
  RollingBack11/1 -> AccOverride/1  "VSM_AccOverride"
  Switch/1 -> ACCFastExit_b/1  "VSM_ACCFastExit"
  [ACCFastExitConditions] -> Logical Operator4/1
  RollingBack/1 -> [RollingBack]
  ESP_MasterCylindBrakePress/1 -> Compare To Constant33/1
  Compare To Constant25/1 -> TrueDurationTime8/1
  [EngLimpHome] -> Bus Creator/15  "VSM_ACCFastExitCons_EngLimpHome"
  Compare To Constant22/1 -> TrueDurationTime5/1
  Compare To Constant124/1 -> RollingBack12/1
  Compare To Constant27/1 -> Bus Creator1/1  "VSM_ACCSlowExitCons_EspActive400ms"
  [DriveBrakeExit] -> Unit Delay/1, Logical Operator15/1
  Compare To Constant4/1 -> RollingBack2/2
  Gain1/1 -> Add/2
  Compare To Constant50/1 -> Bus Creator2/3  "ACCA_VDCActive"
  [DriverSBR] -> Bus Creator1/7  "VSM_ACCFastExitCons_DriverSBR"
  MATLAB Function/1(ActiveConditionsFulfilled) -> ACCActCondF_b/1  "VSM_ACCActCondF"
  Compare To Constant13/1 -> [BrakeDiskOverHeat]  "BrakeDiskOverHeat"
  Gain/1 -> Compare To Constant2/1
  [ACCSlowExitConditions] -> Logical Operator1/1
  [VehicleSpd] -> Compare To Constant131/1
  Compare To Constant54/1 -> Bus Creator2/7  "ACCA_PTCActive"
  Compare To Constant16/1 -> Switch2/3
  Bus Creator2/1 -> [ActiveCondition], Logical Operator8/1  "ActiveEnable"
  Compare To Constant133/1 -> [ACCError_Inhibit]
  [NoForwardGear] -> Bus Creator/8  "VSM_ACCFastExitCons_NoForwardGear"
  DriverDoorSts_1/1 -> Compare To Constant48/1
  Compare To Constant61/1 -> RollingBack11/1
  Compare To Constant8/1 -> RollingBack4/1
  Compare To Constant116/1 -> Switch2/1
  [ACCError_Inhibit] -> Bus Creator/17  "VSM_ACCFastExitCons_ACCError_Inhibit"
  Compare To Constant75/1 -> Logical Operator28/2
  Compare To Constant10/1 -> Switch4/3
  RollingBack12/1 -> [DrivingModExit]
  TrueDurationTime7/1 -> Compare To Constant30/1
  Compare To Constant117/1 -> Switch3/1
  Compare To Constant123/1 -> RollingBack12/2
  Unit Delay1/1 -> Logical Operator15/4
  [Cancel] -> Unit Delay1/1, Logical Operator15/3
  VehicleSpd/1 -> [VehicleSpd], Gain1/1
  [VehSpdDisable] -> Compare To Constant127/1
  [DrivingModExit] -> Bus Creator/14  "VSM_ACCFastExitCons_DrivingModExit"
  Bus Creator/1 -> ACCFastExitConditions/1, [ACCFastExitConditions]  "ACCFastExit"
  [EngineOff] -> Bus Creator/4  "VSM_ACCFastExitCons_EngineOff"
  AccrPedlPosnDiagc_1/1 -> Compare To Constant61/1
  Compare To Constant36/1 -> RollingBack9/2
  Longctrl_Decel_ReqValue/1 -> Signal Copy/1
  DriverDoorSts/1 -> Compare To Constant14/1
  Compare To Constant15/1 -> TrueDurationTime20/1
  RollingBack3/1 -> [DriveBrakeExit]  "DriverBrakeExit"
  BTCActive/1 -> Compare To Constant26/1
  Compare To Constant38/1 -> [ACCOverride15min]
  RollingBack13/1 -> ACCDecEnableBOM/1
  [RollingBack] -> Bus Creator/3  "VSM_ACCFastExitCons_RollingBack"
  Unit Delay/1 -> Logical Operator15/2
  [DriveBrake] -> RollingBack3/1
  RollingBack8/1 -> DriverBrake/1, [DriveBrake]  "VSM_ACC_DriverBrake"
  Switch2/1 -> [DriverDoorOpen]  "DriverDoorOpen"
  Compare To Constant122/1 -> RollingBack12/3
  Compare To Constant130/1 -> RollingBack13/2
  Logical Operator28/1 -> Switch2/2, Switch3/2
  Logical Operator15/1 -> ACC_DriverCancel/1
  EPBSts/1 -> Compare To Constant4/1, Compare To Constant5/1
  DrivingModDis/1 -> Compare To Constant123/1, Compare To Constant122/1, Compare To Constant124/1
  [VehicleSpdDisplay] -> Compare To Constant126/1, Compare To Constant125/1
  Compare To Constant129/1 -> RollingBack13/1
  ECM_ACC_CancelSw/1 -> Compare To Constant74/1
  Compare To Constant19/1 -> [VehicleStandStill]
  HDCControl/1 -> Compare To Constant23/1
  Compare To Constant118/1 -> Switch3/3
  Compare To Constant17/1 -> [APSGuidance]
  [AEBTrigger] -> Bus Creator/12  "VSM_ACCFastExitCons_AEBTrigger"
  Compare To Constant35/1 -> RollingBack8/2
  [VehSpdExit] -> Bus Creator/13  "VSM_ACCFastExitCons_VehSpdExit"
  StandstillNoBrakeForce/1(Out1) -> [StandstillNoBrakeForce]  "StandstillNoBrakeForce"
  AccrPedlPosnDiagc/1 -> Compare To Constant7/1, Compare To Constant36/1
  Compare To Constant127/1 -> Bus Creator2/9  "ACCA_VehSpd"
  Logical Operator1/1 -> Switch1/3
  TrueDurationTime20/1 -> Compare To Constant117/1, Compare To Constant118/1
  axvRefMs2/1 -> Compare To Constant129/1
  AVHSts/1 -> Compare To Constant73/1
  Compare To Constant131/1 -> RollingBack13/3
  [ACCSlowExitConditions] -> Logical Operator10/1
  RollingBack5/1 -> [EngineOff]  "EngineOff"
  VxvRef/1 -> StandstillNoBrakeForce/3(VxvRef)
  Compare To Constant132/1 -> ACCDecDisableBOM/1  "VSM_ACC_BOMExit"
  ACCError/1 -> [ACCError], Compare To Constant133/1  "VSM_Diagnostic_ACCError"
  Compare To Constant7/1 -> RollingBack9/1
  Compare To Constant6/1 -> RollingBack1/1
  Compare To Constant5/1 -> RollingBack2/1
  Compare To Constant30/1 -> Bus Creator1/4  "VSM_ACCSlowExitCons_ABSactive400ms"
  EPB_SwtichPositon/1 -> Compare To Constant6/1
  RollingBack1/1 -> RollingBack2/3
  RLWheelDriveDirection/1 -> Compare To Constant/1
  Sum/1 -> Gain/1
  Compare To Constant32/1 -> Bus Creator1/6  "VSM_ACCSlowExitCons_TCS2active3000ms"
  RollingBack2/1 -> [EPBClosed]  "EPBClosed"
  Compare To Constant29/1 -> Bus Creator1/3  "VSM_ACCSlowExitCons_HDCactive40ms"
  RRWheelSpd/1 -> Sum/2
  BrakeDiskOverHeat/1 -> Compare To Constant13/1
  Compare To Constant1/1 -> RollingBack/4
  Compare To Constant2/1 -> RollingBack/2
  Compare To Constant/1 -> RollingBack/3
  Compare To Constant12/1 -> [EspOff]  "EspOff"
  Start_Stop_Sts_G/1 -> Compare To Constant11/1, Compare To Constant40/1, Compare To Constant41/1, Compare To Constant42/1, Compare To Constant39/1
  DriverSBR/1 -> Compare To Constant15/1
  PTCActive/1 -> Compare To Constant25/1
  Compare To Constant14/1 -> TrueDurationTime2/1
  RollingBack4/1 -> [NoForwardGear]  "NoForwardGear"
  MSRActive/1 -> Compare To Constant22/1
  RollingBack7/1 -> RollingBack8/1
  ABSActive/1 -> Compare To Constant24/1
  EngState/1 -> Compare To Constant10/1
  RollingBack9/1 -> AccPedalTouch/1  "VSM_ACC_AccPedalTouch"
  TrueDurationTime1/1 -> Compare To Constant35/1
  [VehicleStandStill] -> MATLAB Function/2(VehicleStandstill)  "VSM_VehicleStandStill"
  Compare To Constant20/1 -> [Standstill3min]  "Standstill3min"
  ABSActive_1/1 -> Compare To Constant53/1
  DriverSBR_1/1 -> Compare To Constant49/1
  [EspOff] -> Bus Creator/7  "VSM_ACCFastExitCons_EspOff"
  Bus Creator1/1 -> ACCSlowExitConditions/1, [ACCSlowExitConditions]  "ACCSlowExit"
  Logical Operator2/1 -> Switch/1
  [VehicleStandStill] -> StandstillNoBrakeForce/2(VehicleStandstill)
  Compare To Constant53/1 -> Bus Creator2/6  "ACCA_ABSActive"
  Compare To Constant33/1 -> RollingBack7/1
  [TJAActive_b] -> Switch/2
  MSRActive_1/1 -> Compare To Constant51/1
  HDCControl_1/1 -> Compare To Constant52/1
  [TJAActive_b] -> Switch1/2
  Switch1/1 -> ACCSlowExit_b/1  "VSM_ACCSlowExit"
  Compare To Constant48/1 -> Bus Creator2/1  "ACCA_DriverDoorSts"
  PTCActive_1/1 -> Compare To Constant54/1
  Logical Operator3/1 -> Switch/3
  Compare To Constant51/1 -> Bus Creator2/4  "ACCA_MSRActive"
  Compare To Constant52/1 -> Bus Creator2/5  "ACCA_HDCControl"
  Bus Selector/2 -> Logical Operator2/2  "<VSM_ACCFastExitCons_StandstillNoBrakeForce>"
  Bus Selector/4 -> Logical Operator2/4  "<VSM_ACCFastExitCons_EngineOff>"
  Bus Selector/5 -> Logical Operator2/5  "<VSM_ACCFastExitCons_BrakeDiskOverHeat>"
  Bus Selector/6 -> Logical Operator2/6  "<VSM_ACCFastExitCons_Cancel>"
  Compare To Constant49/1 -> Bus Creator2/2  "ACCA_DriverSBR"
  [DriveBrakeExit] -> Bus Creator/9  "VSM_ACCFastExitCons_DriveBrakeExit"
  TrueDurationTime9/1 -> Compare To Constant32/1
  [EPBClosed] -> Bus Creator/10  "VSM_ACCFastExitCons_EPBClosed"
  [DriverDoorOpen] -> Bus Creator/11  "VSM_ACCFastExitCons_DriverDoorOpen"
  Switch5/1 -> Compare To Constant8/1, Compare To Constant9/1
  Bus Selector/1 -> Logical Operator2/1  "<VSM_ACCFastExitCons_Standstill3min>"
  [StandstillNoBrakeForce] -> Bus Creator/2  "VSM_ACCFastExitCons_StandstillNoBrakeForce"
  [BrakeDiskOverHeat] -> Bus Creator/5  "VSM_ACCFastExitCons_BrakeDiskOverHeat"
  AccPedalOverride/1 -> RollingBack11/2
  Compare To Constant74/1 -> [Cancel]  "Cancel"
  Switch3/1 -> [DriverSBR]  "DriverSBR"
  Compare To Constant73/1 -> Logical Operator14/1
  TrueDurationTime6/1 -> Compare To Constant29/1
  Switch6/1 -> Compare To Constant34/1
  [DriveBrake] -> Logical Operator14/2
  Compare To Constant24/1 -> TrueDurationTime7/1
  RLWheelSpd/1 -> Sum/1
  VDCActive_1/1 -> Compare To Constant50/1
  TrueDurationTime5/1 -> Compare To Constant28/1
  VDCActive/1 -> Compare To Constant21/1
  [Cancel] -> Bus Creator/6  "VSM_ACCFastExitCons_Cancel"
  Compare To Constant21/1 -> TrueDurationTime4/1
  RRWheelDriveDirection/1 -> Compare To Constant1/1
  Logical Operator10/1 -> Bus Creator2/11
  RollingBack10/1 -> MATLAB Function/3(ActiveEnable)  "VSM_ActiveEnable"
  Compare To Constant23/1 -> TrueDurationTime6/1
  Compare To Constant28/1 -> Bus Creator1/2  "VSM_ACCSlowExitCons_MSRactive800ms"
  Compare To Constant18/1 -> [AEBTrigger]  "AEB_Trigger"
  AEB_Trigger/1 -> Compare To Constant18/1
  Subsystem/1(Outport) -> ACCDataClct_ConNotStsf/1  "ACCDataClct_ConNotStsf"
  Logical Operator6/1 -> ACCDataClct_OverrideACCExit/1  "ACCDataClct_OverrideACCExit"
  Logical Operator7/1 -> ACCDataClct_DriverBrakeACCExit/1  "ACCDataClct_DriverBrakeACCExit"
  Constant1/1 -> ACCDataClct_DriverSteerACCExit/1  "ACCDataClct_DriverSteerACCExit"
  [ACCMode] -> Compare To Constant37/1
  Compare To Constant37/1 -> TrueDurationTime3/1
  [ACCMode] -> Exit100ms/1(ACCSts)
  Exit100ms/1(Out1) -> Logical Operator7/1, Logical Operator6/2
  [ACCOverride15min] -> Logical Operator6/1
  [DriveBrakeExit] -> Logical Operator7/2
  Logical Operator8/1 -> RollingBack10/1  "ActiveEnable"
  User_ACCSet/1 -> Subsystem/1(User_ACCSet)
  User_Res/1 -> Subsystem/2(User_Res)
  [ACCFastExitConditions] -> Subsystem/3(ACCFastExitConditions)
  [ActiveCondition] -> Subsystem/4(ActiveCondition)
  [ACCMode] -> Subsystem/5(ACCMode)
  ? -> TJADataClct_ConNotStsf/1  "TJADataClct_ConNotStsf"
  HCU_PowertrainSts/1 -> Compare To Constant56/1
  Compare To Constant56/1 -> Switch4/1
  Switch4/1 -> RollingBack5/1
  TGS_Lever/1 -> Switch5/3
  HCU_GearSts/1 -> Switch5/1
  Constant5/1 -> Switch5/2
  Constant7/1 -> Switch4/2
  BrakePedalStatus_G/1 -> Switch6/3
  ConfigiBooster/1 -> Switch6/2
  IB_BrkPedalAppld/1 -> Switch6/1
